simulink library "dynamic_load_lib"  (R2016b)
settings: Solver=ode45  StartTime=0.0  StopTime=10.0  RelTol=1e-3  EnableMultiTasking=on
undefined symbols (not defined in the file): DiscIntNeverNeededParam, Tau, Ts
libraries: powerlib x9, dynamic_load_lib x1, powerlib_meascontrol x1
settings Model: Creator=re25624  LastModifiedBy=jlesage
settings DataIOCC: LimitDataPoints=on  SaveFormat=Array  SignalLoggingSaveFormat=ModelDataLogs
settings OptimizationCC: ExpressionDepthLimit=2147483647  LifeSpan=inf
settings DebuggingCC: UnderspecifiedInitializationDetection=Classic  MergeDetectMultiDrivingBlocksExec=none  SolverPrmCheckMsg=warning  FcnCallInpInsideContextMsg=warning  StateNameClashWarn=warning  SFUnexpectedBacktrackingDiag=warning  SFNoUnconditionalDefaultTransitionDiag=warning  SFExecutionAtInitializationDiag=none
settings HardwareCC: ProdBitPerPointer=32  ProdBitPerSizeT=32  ProdBitPerPtrDiffT=32  ProdLargestAtomicFloat=None  ProdIntDivRoundTo=Undefined  ProdEndianess=Unspecified  ProdWordSize=32  ProdHWDeviceType=32-bit Generic
settings ModelReferenceCC: PropagateSignalLabelsOutOfModel=off
settings GRTTargetCC: TargetLangStandard=C89/C90 (ANSI)  GeneratePreprocessorConditionals=Disable all  CombineOutputUpdateFcns=off  GRTInterface=on
settings ConfigComp: CovMetricSettings=dw  CovHtmlReporting=on  CovSaveCumulativeToWorkspaceVar=on  CovSaveSingleToWorkspaceVar=on  CovExternalEMLEnable=off

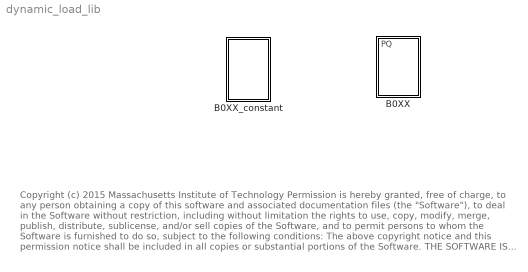
== system dynamic_load_lib ==
  note: Copyright (c) 2015 Massachusetts Institute of Technology
      | Permission is hereby granted, free of charge, to any person obtaining a copy of this software and associated documentation files (the "Software"), to deal in the Software without restriction, including without limitation the rights to use, copy, modify, merge, publish, distribute, sublicense, and/or sell copies of the Software, and to permit persons to whom the Software is furnished to do so, subject to the following conditions:
      |
      | The above copyright notice and this permission notice shall be included in all copies or substantial portions of the Software.
      |
      | THE SOFTWARE IS PROVIDED "AS IS", WITHOUT WARRANTY OF ANY KIND, EXPRESS OR IMPLIED, INCLUDING BUT NOT LIMITED TO THE WARRANTIES OF MERCHANTABILITY, FITNESS FOR A PARTICULAR PURPOSE AND NONINFRINGEMENT. IN NO EVENT SHALL THE AUTHORS OR COPYRIGHT HOLDERS BE LIABLE FOR ANY CLAIM,
      | DAMAGES OR OTHER LIABILITY, WHETHER IN AN ACTION OF CONTRACT, TORT OR OTHERWISE, ARISING FROM, OUT OF OR IN CONNECTION WITH THE SOFTWARE OR THE USE OR OTHER DEALINGS IN THE SOFTWARE.
  B0XX : Subsystem  mask(Dynamic load){V=460, P_Scale=2, Q_Scale=2}
      mask prompts: V "VRMSLL"
      mask help:
      | The dynamic load model is based on three independent current drains (initialized using nominal voltage) following a terminal voltage and the feed-in kW and kVAr.
      |
      | The model was designed to have scale factors for active and reactive power independently (both factors initialized to 1).
      |
      | The current drain of each phase is computed independently permitting unbalanced conditions in the system resulting in unbalanced consumption.
      mask TypeOptions P_Scale: P_Scale/Gain
      mask TypeOptions Q_Scale: Q_Scale/Gain
  B0XX_constant : Subsystem  mask(Static PQ Load){v=460, kVA=100, pf=0.90}
      mask prompts: v "VRMSLL"
      mask help: The static load model is based on the default Simulink parallel load model. However, a mask was created to permit parametrization using nominal voltage, apparent power, and power factor.

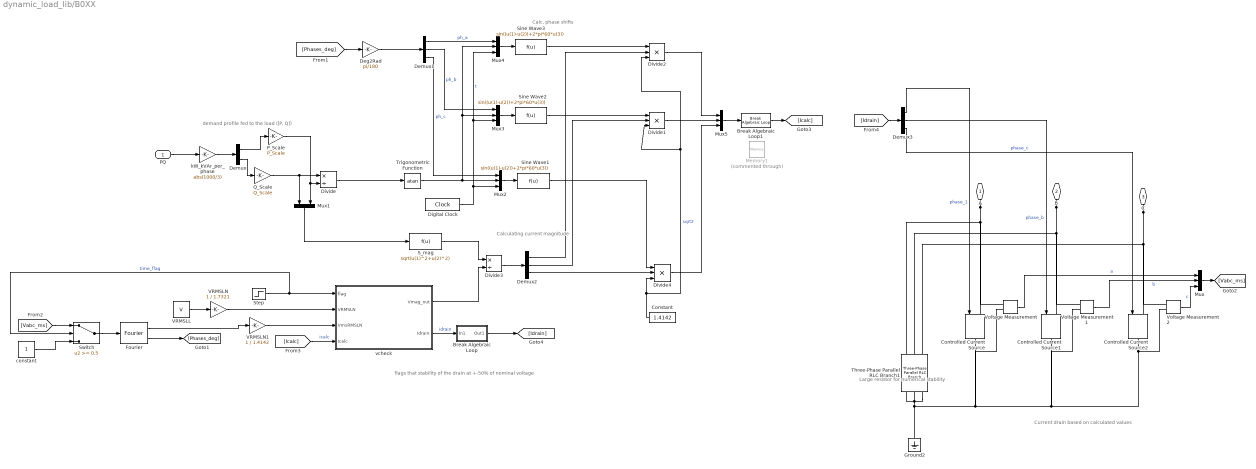
== system dynamic_load_lib/B0XX ==
  note: flags that stability of the drain at +-50% of nominal voltage
  note: Large resistor for numerical stability
  note: Current drain based on calculated values
  note: demand profile fed to the load ([P, Q])
  note: Calculating current magnitude
  note: Calc. phase shifts
  PQ : Inport
  Break Algebraic Loop : Subsystem  mask{Tau=Tau, Ts=Ts}
      mask prompts: Tau "Time Constant"; Ts "Sample Time"
  Break Algebraic Loop1 : dynamic_load_lib/B0XX/Break Algebraic Loop  Tau=Tau  Ts=Ts
  Constant : Constant  Value=1.4142
  Controlled Current Source : powerlib/Electrical Sources/Controlled Current Source  Initialize=on  Source_Type=AC  Amplitude=0  Phase=0  Frequency=0  Measurements=None
  Controlled Current Source1 : powerlib/Electrical Sources/Controlled Current Source  Initialize=on  Source_Type=AC  Amplitude=0  Phase=0  Frequency=0  Measurements=None
  Controlled Current Source2 : powerlib/Electrical Sources/Controlled Current Source  Initialize=on  Source_Type=AC  Amplitude=0  Phase=0  Frequency=0  Measurements=None
  Deg2Rad : Gain  Gain=pi/180
  Demux : Demux  Outputs=2
  Demux1 : Demux  Outputs=3
  Demux2 : Demux  Outputs=3
  Demux3 : Demux  Outputs=3
  Digital Clock : DigitalClock  SampleTime=Ts
  Divide : Product  Inputs=*/
  Divide1 : Product  Inputs=***
  Divide2 : Product  Inputs=***
  Divide3 : Product  Inputs=*/
  Divide4 : Product  Inputs=***
  Fourier : powerlib_meascontrol/Measurements/Fourier  Freq=60  n=1  InInit=[0, 0]  Ts=Ts
  Ground2 : powerlib/Elements/Ground  LConnTagsString=a
  Memory1 : Memory  Commented=through
  Mux{,2..5} (5 alike) : Mux  Inputs=3
  Mux1 : Mux  Inputs=2
  P_Scale : Gain  Gain=P_Scale
  Q_Scale : Gain  Gain=Q_Scale
  S_mag : Fcn  Expr=sqrt(u(1)^2+u(2)^2)
  Sine Wave1 : Fcn  Expr=sin((u(1)-u(2))+2*pi*60*u(3))
  Sine Wave2 : Fcn  Expr=sin((u(1)-u(2))+2*pi*60*u(3))
  Sine Wave3 : Fcn  Expr=sin((u(1)-u(2))+2*pi*60*u(3))
  Step : Step  Time=0.02  SampleTime=Ts
  Switch : Switch  Threshold=0.5
  Three-Phase Parallel RLC Branch1 : powerlib/Elements/Three-Phase Parallel RLC Branch  LConnTagsString=A|B|C  RConnTagsString=A|B|C  BranchType=RLC  Resistance=1e6  Inductance=inf  Capacitance=0  Measurements=None
  Trigonometric Function : Trigonometry  Operator=atan
  VRMSLL : Constant  Value=V
  VRMSLN : Gain  Gain=1 / 1.7321
  VRMSLN1 : Gain  Gain=1 / 1.4142
  Voltage Measurement : powerlib/Measurements/Voltage Measurement  PhasorSimulation=off  OutputType=Complex  PSBequivalent=0
  Voltage Measurement1 : powerlib/Measurements/Voltage Measurement  PhasorSimulation=off  OutputType=Complex  PSBequivalent=0
  Voltage Measurement2 : powerlib/Measurements/Voltage Measurement  PhasorSimulation=off  OutputType=Complex  PSBequivalent=0
  constant : Constant
  kW_kVAr_per_phase : Gain  Gain=abs(1000/3)
  vcheck : MATLAB Function  TreatAsAtomicUnit=on  SystemSampleTime=Ts
  A : PMIOPort  Port=1  Side=Left
  B : PMIOPort  Port=2  Side=Left
  C : PMIOPort  Port=3  Side=Left
  wires:
  kW_kVAr_per_phase/1 -> Demux/1
  Demux/1 -> P_Scale/1
  Demux/2 -> Q_Scale/1
  Q_Scale/1 -> Divide/1, Mux1/1
  P_Scale/1 -> Divide/2, Mux1/2
  Divide/1 -> Trigonometric Function/1
  Trigonometric Function/1 -> Mux3/2, Mux4/2, Mux2/2
  Mux1/1 -> S_mag/1
  S_mag/1 -> Divide3/1
  Constant/1 -> Divide2/3, Divide1/3, Divide4/3  "sqrt2"
  Mux2/1 -> Sine Wave1/1
  Sine Wave1/1 -> Divide4/1
  Digital Clock/1 -> Mux4/3, Mux3/3, Mux2/3  "t"
  [Phases_deg] -> Deg2Rad/1
  Voltage Measurement/1 -> Mux/1  "a"
  Voltage Measurement1/1 -> Mux/2  "b"
  Voltage Measurement2/1 -> Mux/3  "c"
  Mux/1 -> [Vabc_ms]
  Mux3/1 -> Sine Wave2/1
  Mux4/1 -> Sine Wave3/1
  Demux1/1 -> Mux4/1  "ph_a"
  Demux1/2 -> Mux3/1  "ph_b"
  Demux1/3 -> Mux2/1  "ph_c"
  Sine Wave3/1 -> Divide2/1
  Sine Wave2/1 -> Divide1/1
  Step/1 -> vcheck/1(flag), Switch/2  "time_flag"
  Fourier/1 -> VRMSLN1/1
  vcheck/1(Vmag_out) -> Divide3/2
  Divide3/1 -> Demux2/1
  Demux2/1 -> Divide2/2
  Demux2/2 -> Divide1/2
  Demux2/3 -> Divide4/2
  Divide2/1 -> Mux5/1
  Divide1/1 -> Mux5/2
  Divide4/1 -> Mux5/3
  Demux3/1 -> Controlled Current Source/1  "phase_1"
  Demux3/2 -> Controlled Current Source1/1  "phase_b"
  Demux3/3 -> Controlled Current Source2/1  "phase_c"
  [Icalc] -> vcheck/4(Icalc)  "icalc"
  vcheck/2(Idrain) -> Break Algebraic Loop/1(In1)  "idrain"
  [Idrain] -> Demux3/1
  VRMSLN/1 -> vcheck/2(VRMSLN)
  VRMSLN1/1 -> vcheck/3(VmsRMSLN)
  Break Algebraic Loop/1(Out1) -> [Idrain]
  Deg2Rad/1 -> Demux1/1
  VRMSLL/1 -> VRMSLN/1
  Fourier/2 -> [Phases_deg]
  Switch/1 -> Fourier/1
  [Vabc_ms] -> Switch/1
  constant/1 -> Switch/3
  PQ/1 -> kW_kVAr_per_phase/1
  Mux5/1 -> Break Algebraic Loop1/1
  Break Algebraic Loop1/1 -> [Icalc]
  connections:
  A/RConn1 -- Three-Phase Parallel RLC Branch1/RConn1 -- Voltage Measurement/LConn1 -- Controlled Current Source/LConn1
  B/RConn1 -- Three-Phase Parallel RLC Branch1/RConn2 -- Voltage Measurement1/LConn1 -- Controlled Current Source1/LConn1
  C/RConn1 -- Three-Phase Parallel RLC Branch1/RConn3 -- Voltage Measurement2/LConn1 -- Controlled Current Source2/LConn1
  Voltage Measurement2/LConn2 -- Controlled Current Source2/RConn1 -- Three-Phase Parallel RLC Branch1/LConn1 -- Three-Phase Parallel RLC Branch1/LConn2 -- Three-Phase Parallel RLC Branch1/LConn3 -- Ground2/LConn1 -- Voltage Measurement/LConn2 -- Controlled Current Source/RConn1 -- Voltage Measurement1/LConn2 -- Controlled Current Source1/RConn1

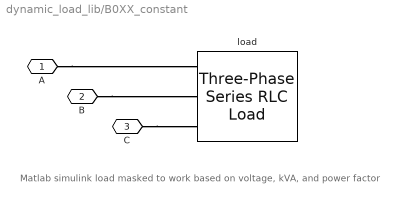
== system dynamic_load_lib/B0XX_constant ==
  note: Matlab simulink load masked to work based on voltage, kVA, and power factor
  load : powerlib/Elements/Three-Phase Series RLC Load  LConnTagsString=A|B|C  Configuration=Y (grounded)  NominalVoltage=v  Vabc=[1e3 1e3 1e3]  Vabcp=[1e3 1e3 1e3]  NominalFrequency=60  UnbalancedPower=off  ActivePower=kVA*1E3*pf  InductivePower=kVA*1E3*sqrt(1-pf^2)  CapacitivePower=0  Pabc=[10e3 9e3 11e3]  QLabc=[100 90 110]  QCabc=[100 90 110]  Pabcp=[10e3 9e3 11e3]  QLabcp=[100 90 110]  QCabcp=[100 90 110]  Measurements=None  LoadType=constant Z
  A : PMIOPort  Port=1  Side=Left
  B : PMIOPort  Port=2  Side=Left
  C : PMIOPort  Port=3  Side=Left
  connections:
  C/RConn1 -- load/LConn3
  B/RConn1 -- load/LConn2
  A/RConn1 -- load/LConn1

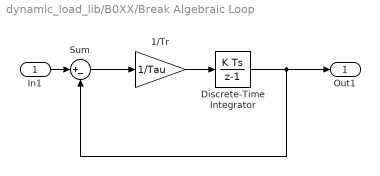
== system dynamic_load_lib/B0XX/Break Algebraic Loop ==
  In1 : Inport
  1/Tr : Gain  Gain=1/Tau  SampleTime=Ts
  Discrete-Time Integrator : DiscreteIntegrator  SampleTime=Ts  ICPrevOutput=DiscIntNeverNeededParam  ICPrevScaledInput=DiscIntNeverNeededParam
  Sum : Sum  Inputs=|+-
  Out1 : Outport
  wires:
  In1/1 -> Sum/1
  Discrete-Time Integrator/1 -> Out1/1, Sum/2
  1/Tr/1 -> Discrete-Time Integrator/1
  Sum/1 -> 1/Tr/1

== matlab function dynamic_load_lib/B0XX/vcheck ==
  data: flag input; Vmag_out output; VRMSLN input; VmsRMSLN input; Idrain output; Icalc input
function [Vmag_out,Idrain] = vcheck(flag, VRMSLN, VmsRMSLN, Icalc)
%#codegen
% stability_flag at +-50% of nominal voltage
disable = (sum(VmsRMSLN>VRMSLN*1.5)>0)||(sum(VmsRMSLN<VRMSLN*0.5)>0);

if flag==0
    
    Vmag_out = [VRMSLN; VRMSLN; VRMSLN];
    % elseif stability_flag
    %     Vmag_out = [0; 0; 0];
else
    Vmag_out = VmsRMSLN;
end

if disable==1
    Idrain = [0;0;0];
else
    Idrain = Icalc;
end
